simulink model "graficas"  (R2017b)
settings: Solver=FixedStepAuto  StartTime=0.0  StopTime=10.0  FixedStep=0.001  RelTol=1e-3
libraries: cstblocks x4
settings Model: Creator=Enrique  LastModifiedBy=Enrique

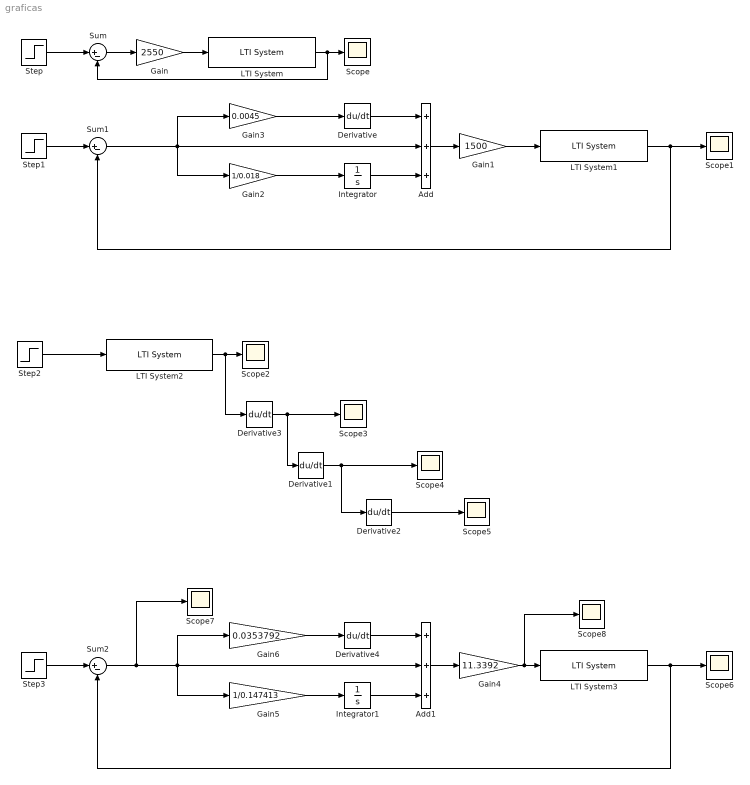
== system graficas ==
  Add : Sum  Inputs=+++
  Add1 : Sum  Inputs=+++
  Derivative{,1..4} (5 alike) : Derivative
  Gain : Gain  Gain=2550
  Gain1 : Gain  Gain=1500
  Gain2 : Gain  Gain=1/0.018
  Gain3 : Gain  Gain=0.0045
  Gain4 : Gain  Gain=11.3392
  Gain5 : Gain  Gain=1/0.147413
  Gain6 : Gain  Gain=0.0353792
  Integrator : Integrator
  Integrator1 : Integrator
  LTI System : cstblocks/LTI System  sys=sys_2  IC=[]
  LTI System1 : cstblocks/LTI System  sys=sys_2  IC=[]
  LTI System2 : cstblocks/LTI System  sys=sys_1  IC=[]
  LTI System3 : cstblocks/LTI System  sys=sys_1  IC=[]
  Scope{,1..8} (9 alike) : Scope
  Step{,1..3} (4 alike) : Step  Time=0  SampleTime=0
  Sum : Sum  Inputs=|+-
  Sum1 : Sum  Inputs=|+-
  Sum2 : Sum  Inputs=|+-
  wires:
  Gain/1 -> LTI System/1
  Sum/1 -> Gain/1
  Step/1 -> Sum/1
  LTI System/1 -> Scope/1, Sum/2
  LTI System1/1 -> Scope1/1, Sum1/2
  Step1/1 -> Sum1/1
  Sum1/1 -> Gain2/1, Gain3/1, Add/2
  Add/1 -> Gain1/1
  Gain1/1 -> LTI System1/1
  Gain2/1 -> Integrator/1
  Gain3/1 -> Derivative/1
  Derivative/1 -> Add/1
  Integrator/1 -> Add/3
  LTI System2/1 -> Derivative3/1, Scope2/1
  Step2/1 -> LTI System2/1
  Derivative2/1 -> Scope5/1
  Derivative1/1 -> Derivative2/1, Scope4/1
  Derivative3/1 -> Derivative1/1, Scope3/1
  LTI System3/1 -> Scope6/1, Sum2/2
  Step3/1 -> Sum2/1
  Gain5/1 -> Integrator1/1
  Gain6/1 -> Derivative4/1
  Sum2/1 -> Scope7/1, Gain5/1, Gain6/1, Add1/2
  Gain4/1 -> Scope8/1, LTI System3/1
  Add1/1 -> Gain4/1
  Integrator1/1 -> Add1/3
  Derivative4/1 -> Add1/1
